simulink model "Project"  (R2019b)
settings: Solver=VariableStepAuto  StartTime=0.0  StopTime=1000  RelTol=1e-3
libraries: simulink x1
(part 1 of 2)
settings Model: Creator=Denis  LastModifiedBy=Denis
settings SolverCC: MaxConsecutiveMinStep=3

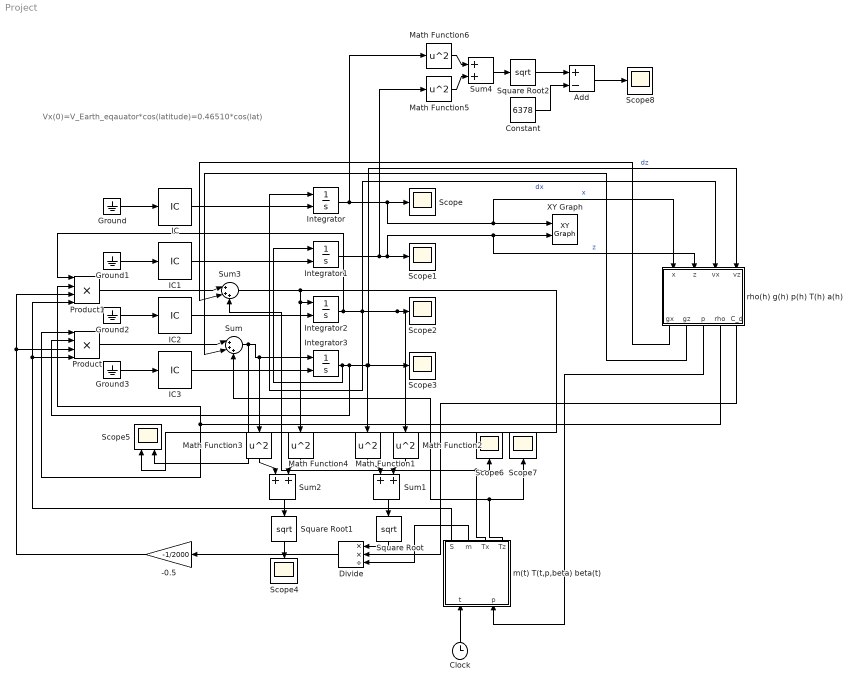
== system Project ==
  note: Vx(0)=V_Earth_eqauator*cos(latitude)=0.46510*cos(lat)
  -0.5 : Gain  Gain=-1/2000
  Add : Sum  Inputs=+-
  Clock : Clock
  Constant : Constant  Value=6378
  Divide : Product  Inputs=**/
  Ground{,1..3} (4 alike) : Ground
  IC : InitialCondition  Value=0
  IC1 : InitialCondition  Value=6378
  IC2 : InitialCondition  Value=0
  IC3 : InitialCondition  Value=0
  Integrator{,1..3} (4 alike) : Integrator  InitialConditionSource=external
  Math Function{1..6} (6 alike) : Math  Operator=square  SignedPower=off  SaturateOnIntegerOverflow=on
  Product : Product  Inputs=4
  Product1 : Product  Inputs=4
  Scope{,1..4,6..8} (8 alike) : Scope
  Scope5 : Scope  NumInputPorts=2
  Square Root : Sqrt  SaturateOnIntegerOverflow=on
  Square Root1 : Sqrt  SaturateOnIntegerOverflow=on
  Square Root2 : Sqrt  SaturateOnIntegerOverflow=on
  Sum : Sum  Inputs=|+++
  Sum1 : Sum
  Sum2 : Sum
  Sum3 : Sum  Inputs=|+++
  Sum4 : Sum
  XY Graph : simulink/Sinks/XY Graph  xmin=-7500  xmax=7500  ymin=-7500  ymax=7500  st=0.1
  m(t) T(t,p,beta) beta(t) : MATLAB Function  TreatAsAtomicUnit=on
  rho(h) g(h) p(h) T(h) a(h) : MATLAB Function  TreatAsAtomicUnit=on
  wires:
  Ground/1 -> IC/1
  Ground1/1 -> IC1/1
  Ground2/1 -> IC2/1
  Ground3/1 -> IC3/1
  IC3/1 -> Integrator3/2
  IC2/1 -> Integrator2/2
  IC1/1 -> Integrator1/2
  IC/1 -> Integrator/2
  Integrator/1 -> Math Function6/1, XY Graph/1, rho(h) g(h) p(h) T(h) a(h)/1(x), Scope/1  "x"
  Integrator1/1 -> Math Function5/1, rho(h) g(h) p(h) T(h) a(h)/2(z), XY Graph/2, Scope1/1  "z"
  Integrator2/1 -> Product1/1, rho(h) g(h) p(h) T(h) a(h)/3(vx), Math Function2/1, Scope2/1, Integrator/1  "dx"
  Integrator3/1 -> Product/2, rho(h) g(h) p(h) T(h) a(h)/4(vz), Scope3/1, Math Function1/1, Integrator1/1  "dz"
  Sum/1 -> Scope5/2, Integrator3/1, Math Function3/1
  Product/1 -> Sum/1
  -0.5/1 -> Product/3, Product1/3
  Product1/1 -> Sum3/1
  rho(h) g(h) p(h) T(h) a(h)/4(rho) -> Product1/2, Product/1
  Math Function1/1 -> Sum1/1
  Math Function2/1 -> Sum1/2
  Sum1/1 -> Square Root/1
  Sum2/1 -> Square Root1/1
  Math Function4/1 -> Sum2/2
  Math Function3/1 -> Sum2/1
  Square Root1/1 -> Scope4/1
  Divide/1 -> -0.5/1
  rho(h) g(h) p(h) T(h) a(h)/1(gx) -> Sum3/2
  Sum3/1 -> Scope5/1, Math Function4/1, Integrator2/1
  rho(h) g(h) p(h) T(h) a(h)/2(gz) -> Sum/2
  Clock/1 -> m(t) T(t,p,beta) beta(t)/1(t)
  Square Root/1 -> Divide/1
  m(t) T(t,p,beta) beta(t)/1(S) -> Product1/4, Product/4
  m(t) T(t,p,beta) beta(t)/3(Tx) -> Scope6/1, Sum3/3
  m(t) T(t,p,beta) beta(t)/4(Tz) -> Scope7/1, Sum/3
  rho(h) g(h) p(h) T(h) a(h)/3(p) -> m(t) T(t,p,beta) beta(t)/2(p)
  m(t) T(t,p,beta) beta(t)/2(m) -> Divide/3
  rho(h) g(h) p(h) T(h) a(h)/5(C_d) -> Divide/2
  Square Root2/1 -> Add/1
  Sum4/1 -> Square Root2/1
  Math Function6/1 -> Sum4/1
  Math Function5/1 -> Sum4/2
  Constant/1 -> Add/2
  Add/1 -> Scope8/1

== matlab function Project/m(t) T(t,p,beta) beta(t) ==
  data: S output; t input; m output; Tx output; Tz output; p input
function [S, m, Tx, Tz] = timed(t, p)
%% Initialize mass constants
m_payload = 475;
m_frame = [2717, 544];
m_propellant = [39463, 4037];
m0 = m_payload+m_frame(1)+m_frame(2)+m_propellant(1)+m_propellant(2);
%% Initialize thrust values and subvalues
T = [62.5, 3.2];
T_newton = 9964.016384.*T;
Isp = [304, 325];
g0 = 9.8;
dm = T_newton./(g0.*Isp);
t_burnout = m_propellant./dm;
%% Initialize beta and phase
t_phase = [0,10,20,30,50,75,100,140,175,191.34,193,195,220,260,310,350,390,420,490,560,605];
beta_phase = [90,90,89.973,89.898,84.76,71.349,56.021,38.934,30.622,37.74,37.74,37.74,31.095,26.718,19.356,13.096,6.49,0.758,-10.614,-27.413,-27.413];
%beta_phase = [90,90,89.973,89.898,84.76,73.349,60.021,38.934,34.622,33.74,33.74,33.74,32.095,26.718,19.356,13.096,1.49,0.758,-20.614,-30.413,-40.413];
beta = interp1(t_phase,beta_phase,t);
A_e = [0.9,0.2];
% beta = beta_phase(phase_current-1)+(t-t_phase_current(phase_current-1))/(t_phase_current(phase)-t_phase(phase_current-1))*(beta(phase_current)-beta(phase_current-1)); % Thrust direction angle

%% Calculating S and m from t
if t<t_burnout(1)
    m = m0 - dm(1)*t;
    S = 3.14;
    Tx = (T_newton(1)-A_e(1)*p)*cosd(beta)/(1000*m);
    Tz = (T_newton(1)-A_e(1)*p)*sind(beta)/(1000*m);
elseif t_burnout(1)<=t & t<193
    m = m_payload+m_frame(1)+m_frame(2)+m_propellant(2);
    S = 3.14;
    Tx = 0;
    Tz = 0;
elseif 193<=t & t<195
    m = m_payload+m_frame(2)+m_propellant(2);
    S = 1;
    Tx = 0;
    Tz = 0;
elseif 195<=t & t<195+t_burnout(2)
    m = m_payload+m_frame(2)+m_propellant(2)-dm(2)*(t-195);
    S = 1;
    Tx = (T_newton(2)-A_e(2)*p)*cosd(beta)/(1000*m);
    Tz = (T_newton(2)-A_e(2)*p)*sind(beta)/(1000*m);
elseif 195+t_burnout(2)<=t
    m = m_payload;
    S = 1;
    Tx = 0;
    Tz = 0;
else
    m = m_payload;
    S = 1;
    Tx = 0;
    Tz = 0;
end
